simulink model "linear_acceleration"  (R2024b)
settings: Solver=VariableStepAuto  StartTime=0.0  StopTime=0.6  RelTol=1e-3
values from neighbouring files (symbols this model uses):
  tau = 0.1    [simulate_contouring_error.m]
settings Model: Creator=shohei  LastModifiedBy=shohei

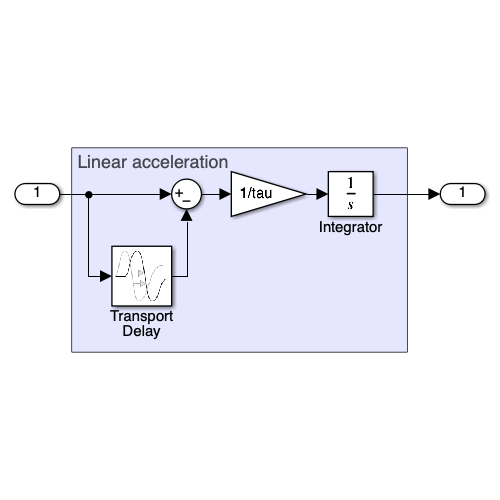
[thumbnail: Simulink's stored preview of the top-level diagram]
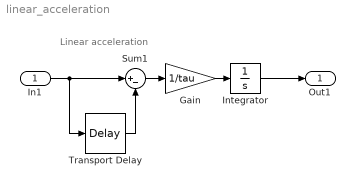
== system linear_acceleration ==
  note: Linear acceleration
  In1 : Inport
  Gain : Gain  Gain=1/tau
  Integrator : Integrator
  Sum1 : Sum  Inputs=|+-
  Transport Delay : TransportDelay  DelayTime=tau  PadeOrder=n
  Out1 : Outport
  wires:
  Sum1/1 -> Gain/1
  In1/1 -> Transport Delay/1, Sum1/1
  Gain/1 -> Integrator/1
  Transport Delay/1 -> Sum1/2
  Integrator/1 -> Out1/1
